simulink model "Vertical_rolling_Tongji_Control"  (R2021b)
settings: Solver=ode23s  StartTime=0.0  StopTime=7.5  FixedStep=1e-3  MaxStep=1e-3  RelTol=1e-3
values from neighbouring files (symbols this model uses):
  J_1 = m_1*r_1^2/2    (= 0.1)    [Vertical_Rolling_Tongji.m]
  J_2 = m_2*r_2^2/2    (= 2.5)    [Vertical_Rolling_Tongji.m]
  Klqr = lqr(sys,transpose(C)*Qu*C,R)    [Vertical_Rolling_Tongji.m]
  m_1 = 5    [Vertical_Rolling_Tongji.m]
  m_2 = 20    [Vertical_Rolling_Tongji.m]
  mu_d = 0.5    [Vertical_Rolling_Tongji.m]
  mu_r = mu_s*10^-2    (= 0.0065)    [Vertical_Rolling_Tongji.m]
  mu_s = 0.65    [Vertical_Rolling_Tongji.m]
  r_1 = 0.2    [Vertical_Rolling_Tongji.m]
  r_2 = 0.5    [Vertical_Rolling_Tongji.m]
  resolution = 5e-3    (= 0.005)    [Vertical_Rolling_Tongji.m]
  theta_1_0 = pi/3    (= 1.0471975512)    [Vertical_Rolling_Tongji.m]
libraries: simulink x1
settings Model: Creator=Gioele  LastModifiedBy=gioele
settings SolverCC: AlgebraicLoopSolver=TrustRegion
settings DebuggingCC: AlgebraicLoopMsg=none  SFMachineParentedDataDiag=warning

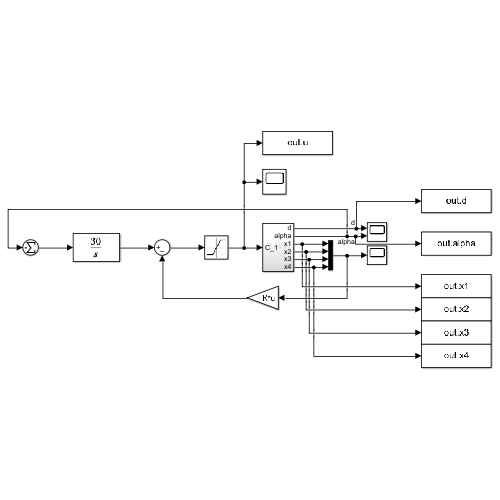
[thumbnail: Simulink's stored preview of the top-level diagram]
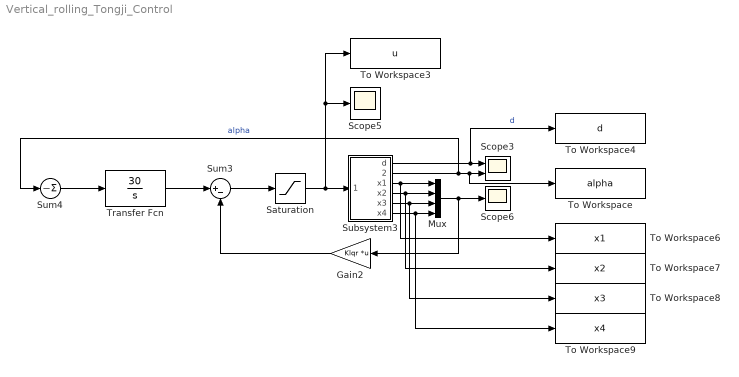
== system Vertical_rolling_Tongji_Control ==
  Gain2 : Gain  Gain=Klqr  Multiplication=Matrix(K*u)
  Mux : Mux
  Saturation : Saturate  UpperLimit=6  LowerLimit=-6
  Scope3 : Scope  NumInputPorts=2
  Scope5 : Scope
  Scope6 : Scope
  Subsystem3 : Subsystem
  Sum3 : Sum  Inputs=|+-
  Sum4 : Sum  Inputs=-
  To Workspace : ToWorkspace  VariableName=alpha  SampleTime=resolution
      settings: Save2DSignal=2-D array (concatenate along first dimension)
  To Workspace3 : ToWorkspace  VariableName=u  SampleTime=resolution
  To Workspace4 : ToWorkspace  VariableName=d  SampleTime=resolution
      settings: Save2DSignal=2-D array (concatenate along first dimension)
  To Workspace6 : ToWorkspace  VariableName=x1  SampleTime=-1
      settings: Save2DSignal=2-D array (concatenate along first dimension)
  To Workspace7 : ToWorkspace  VariableName=x2  SampleTime=-1
      settings: Save2DSignal=2-D array (concatenate along first dimension)
  To Workspace8 : ToWorkspace  VariableName=x3  SampleTime=-1
      settings: Save2DSignal=2-D array (concatenate along first dimension)
  To Workspace9 : ToWorkspace  VariableName=x4  SampleTime=-1
      settings: Save2DSignal=2-D array (concatenate along first dimension)
  Transfer Fcn : TransferFcn  Numerator=[30]  Denominator=[1 0]
  wires:
  Subsystem3/3(x1) -> To Workspace6/1, Mux/1
  Subsystem3/4(x2) -> Mux/2, To Workspace7/1
  Subsystem3/5(x3) -> Mux/3, To Workspace8/1
  Subsystem3/6(x4) -> Mux/4, To Workspace9/1
  Subsystem3/1(d) -> To Workspace4/1, Scope3/1  "d"
  Subsystem3/2(alpha) -> To Workspace/1, Scope3/2, Sum4/1  "alpha"
  Mux/1 -> Scope6/1, Gain2/1
  Gain2/1 -> Sum3/2
  Saturation/1 -> Subsystem3/1(C_1), To Workspace3/1, Scope5/1
  Sum3/1 -> Saturation/1
  Sum4/1 -> Transfer Fcn/1
  Transfer Fcn/1 -> Sum3/1

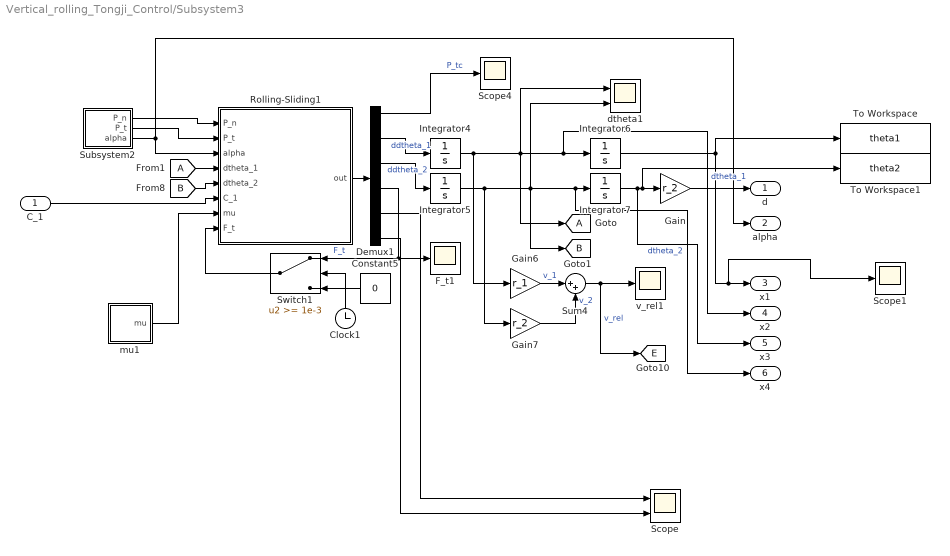
== system Vertical_rolling_Tongji_Control/Subsystem3 ==
  C_1 : Inport
  Clock1 : Clock
  Constant5 : Constant  Value=0
  Demux1 : Demux  Outputs=6
  F_t1 : Scope
  Gain : Gain  Gain=r_2
  Gain6 : Gain  Gain=r_1
  Gain7 : Gain  Gain=r_2
  Integrator4 : Integrator
  Integrator5 : Integrator
  Integrator6 : Integrator  InitialCondition=theta_1_0
  Integrator7 : Integrator
  Rolling-Sliding1 : MATLAB Function  TreatAsAtomicUnit=on
  Scope : Scope  NumInputPorts=2
  Scope1 : Scope
  Scope4 : Scope
  Subsystem2 : Subsystem
  Sum4 : Sum  Inputs=|++
  Switch1 : Switch  Threshold=1e-3  ZeroCross=off
  To Workspace : ToWorkspace  VariableName=theta1  SampleTime=resolution
  To Workspace1 : ToWorkspace  VariableName=theta2  SampleTime=resolution
  dtheta1 : Scope  NumInputPorts=2
  mu1 : Subsystem
  v_rel1 : Scope
  d : Outport
  alpha : Outport  Port=2
  x1 : Outport  Port=3
  x2 : Outport  Port=4
  x3 : Outport  Port=5
  x4 : Outport  Port=6
  tag scope: A=global, B=global, E=global
  wires:
  Subsystem2/2(P_t) -> Rolling-Sliding1/2(P_t)
  Integrator7/1 -> x3/1, To Workspace1/1, Gain/1
  Demux1/4 -> F_t1/1, Switch1/1  "F_t"
  mu1/1(mu) -> Rolling-Sliding1/7(mu)
  Integrator4/1 -> x2/1, Integrator6/1, [A], dtheta1/1, Gain6/1  "dtheta_1"
  Constant5/1 -> Switch1/3
  Gain6/1 -> Sum4/1  "v_1"
  [A] -> Rolling-Sliding1/4(dtheta_1)
  Clock1/1 -> Switch1/2
  Demux1/1 -> Scope4/1  "P_tc"
  Demux1/3 -> Integrator5/1  "ddtheta_2"
  Integrator5/1 -> Integrator7/1, x4/1, [B], dtheta1/2, Gain7/1  "dtheta_2"
  Subsystem2/1(P_n) -> Rolling-Sliding1/1(P_n)
  Demux1/2 -> Integrator4/1  "ddtheta_1"
  Switch1/1 -> Rolling-Sliding1/8(F_t)
  Integrator6/1 -> To Workspace/1, Scope1/1, x1/1
  Gain7/1 -> Sum4/2  "v_2"
  Rolling-Sliding1/1(out) -> Demux1/1
  Sum4/1 -> [E], v_rel1/1  "v_rel"
  [B] -> Rolling-Sliding1/5(dtheta_2)
  C_1/1 -> Rolling-Sliding1/6(C_1)
  Subsystem2/3(alpha) -> Rolling-Sliding1/3(alpha), alpha/1
  Gain/1 -> d/1
  Demux1/5 -> Scope/1
  Demux1/6 -> Scope/2

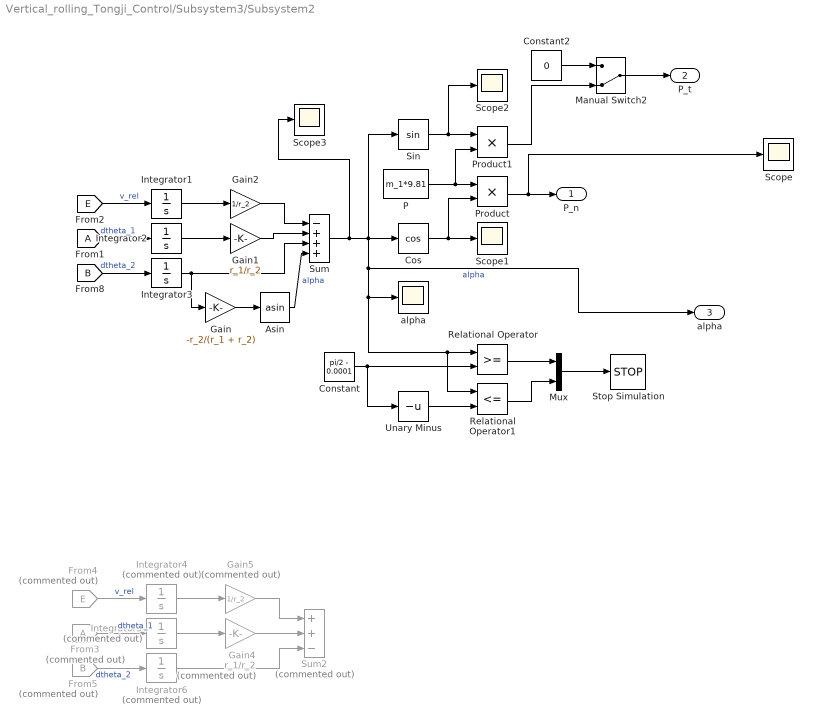
== system Vertical_rolling_Tongji_Control/Subsystem3/Subsystem2 ==
  Asin : Trigonometry  Operator=asin
  Constant : Constant  Value=pi/2 - 0.0001
  Constant2 : Constant  Value=0
  Cos : Trigonometry  Operator=cos
  From3 : From  Commented=on  TagVisibility=global
  From4 : From  Commented=on  GotoTag=E  TagVisibility=global
  From5 : From  Commented=on  GotoTag=B  TagVisibility=global
  Gain : Gain  Gain=-r_2/(r_1 + r_2)
  Gain1 : Gain  Gain=r_1/r_2
  Gain2 : Gain  Gain=1/r_2
  Gain4 : Gain  Commented=on  Gain=r_1/r_2
  Gain5 : Gain  Commented=on  Gain=1/r_2
  Integrator1 : Integrator
  Integrator2 : Integrator  InitialCondition=theta_1_0
  Integrator3 : Integrator
  Integrator4 : Integrator  Commented=on
  Integrator5 : Integrator  Commented=on  InitialCondition=theta_1_0
  Integrator6 : Integrator  Commented=on
  Manual Switch2 : ManualSwitch  CurrentSetting=0
  Mux : Mux  Inputs=2
  P : Constant  Value=m_1*9.81
  Product : Product
  Product1 : Product
  Relational Operator : RelationalOperator  OutDataTypeStr=boolean  RndMeth=Simplest
  Relational Operator1 : RelationalOperator  Operator=<=  OutDataTypeStr=boolean  RndMeth=Simplest
  Scope{,1..3} (4 alike) : Scope
  Sin : Trigonometry
  Stop Simulation : Stop
  Sum : Sum  Inputs=-+++
  Sum2 : Sum  Commented=on  Inputs=++-
  Unary Minus : UnaryMinus
  "alpha " : Scope
  P_n : Outport
  P_t : Outport  Port=2
  alpha : Outport  Port=3
  wires:
  P/1 -> Product1/2, Product/1
  [A] -> Integrator2/1  "dtheta_1"
  Integrator3/1 -> Sum/3, Gain/1
  Integrator2/1 -> Gain1/1
  [B] -> Integrator3/1  "dtheta_2"
  Product/1 -> Scope/1, P_n/1
  Gain1/1 -> Sum/2
  Cos/1 -> Scope1/1, Product/2
  [E] -> Integrator1/1  "v_rel"
  Integrator1/1 -> Gain2/1
  Gain2/1 -> Sum/1
  Constant/1 -> Unary Minus/1, Relational Operator/2
  Unary Minus/1 -> Relational Operator1/2
  Relational Operator/1 -> Mux/1
  Relational Operator1/1 -> Mux/2
  Mux/1 -> Stop Simulation/1
  Sin/1 -> Scope2/1, Product1/1
  Product1/1 -> Manual Switch2/2
  Constant2/1 -> Manual Switch2/1
  Manual Switch2/1 -> P_t/1
  From4/1 -> Integrator4/1  "v_rel"
  Integrator5/1 -> Gain4/1
  From3/1 -> Integrator5/1  "dtheta_1"
  Integrator6/1 -> Sum2/3
  From5/1 -> Integrator6/1  "dtheta_2"
  Gain4/1 -> Sum2/2
  Gain5/1 -> Sum2/1
  Integrator4/1 -> Gain5/1
  Sum/1 -> Scope3/1, Sin/1, Relational Operator1/1, Relational Operator/1, "alpha "/1, alpha/1, Cos/1  "alpha"
  Gain/1 -> Asin/1
  Asin/1 -> Sum/4  "alpha"

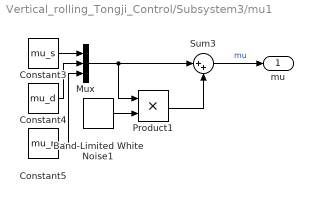
== system Vertical_rolling_Tongji_Control/Subsystem3/mu1 ==
  Band-Limited White Noise1 : simulink/Sources/Band-Limited White Noise  Cov=[0.000001]  Ts=0.1  seed=[23341]
  Constant3 : Constant  Value=mu_s
  Constant4 : Constant  Value=mu_d
  Constant5 : Constant  Value=mu_r
  Mux : Mux  Inputs=3
  Product1 : Product
  Sum3 : Sum  Inputs=|++
  mu : Outport
  wires:
  Sum3/1 -> mu/1  "mu"
  Constant5/1 -> Mux/3
  Constant4/1 -> Mux/2
  Product1/1 -> Sum3/2
  Constant3/1 -> Mux/1
  Mux/1 -> Sum3/1, Product1/1
  Band-Limited White Noise1/1 -> Product1/2

== matlab function Vertical_rolling_Tongji_Control/Subsystem3/Rolling-Sliding1 ==
  data: P_n input; P_t input; alpha input; dtheta_1 input; dtheta_2 input; C_1 input; r_1 parameter; r_2 parameter; J_1 parameter; J_2 parameter; mu input; F_t input; out output; m_2 parameter
function out = fcn(P_n,P_t,alpha,dtheta_1,dtheta_2,C_1,r_1,r_2,J_1,J_2,mu,F_t, m_2)
% Define the inputs of the function, some will be variables coming from the
% system, others will be parametsr from the workspace

mu_s_n = mu(1);
mu_d_n = mu(2);
mu_r_n = mu(3);
% Extract the values for the coefficients of friction from the white noise
% simulator

if abs(dtheta_1) > 0.01
    C_rf1 = - sign(dtheta_1)*mu_r_n*P_n;
else
%     if abs(C_1) < mu_r_n*P_n
%         C_rf1 = - C_1;
%     else
%         C_rf1 = - sign(dtheta_1)*mu_r_n*P_n;
%     end
    C_rf1 = 0;
end
% C_rf1 = - sign(dtheta_1)*mu_r_n*P_n;
if abs(dtheta_2) > 0.01
    C_rf2 = - sign(dtheta_2)*mu_r_n*P_n;
else
%     if abs(- F_t*r_2) < mu_r_n*P_n
%         C_rf2 = - (- F_t*r_2);
%     else
%         C_rf2 = - sign(dtheta_2)*mu_r_n*P_n;
%     end
    C_rf2 = 0;
end
% C_rf2 = - sign(dtheta_2)*mu_r_n*P_n;
% Define the action of the rolling friction forces C_rf1 and C_rf2

if (-0.0001 < dtheta_1*r_1 + dtheta_2*r_2) && (dtheta_1*r_1 + dtheta_2*r_2 < 0.0001)
    % Condition should be (dtheta_1*r_1 + dtheta_2*r_2 == 0) but need
    % tolerance for simulation reasons
    P_tc = P_t;
    F_t = (C_1*(r_1/J_1) + C_rf1*(r_1/J_1) + C_rf2*(r_2/J_2) - P_tc*(r_1^2/J_1) - P_tc*(r_2^2/J_2) - P_n*sin(alpha)*(r_2^2/(J_2+m_2*r_2^2)))/((r_1^2/J_1) + (r_2^2/J_2));
    % Define the two tangential forces P_tc and F_t in the pure rolling
    % case
    if (abs(F_t + P_tc) > mu_s_n*P_n)
        P_tc = sign(alpha)*mu_d_n*P_n;
        F_t = sign(dtheta_1*r_1 + dtheta_2*r_2)*mu_d_n*P_n;
        % Transition from Rolling to Rolling with sliding
    end
else
    P_tc = sign(alpha)*mu_d_n*P_n;
    F_t = sign(dtheta_1*r_1 + dtheta_2*r_2)*mu_d_n*P_n;
    % Define the two tangential forces P_tc and F_t in the pure rolling
    % case
end

ddtheta_1 = (C_1 + C_rf1 - F_t*r_1 - P_tc*r_1)/(J_1);
ddtheta_2 = ((- F_t*r_2 - P_tc*r_2 + C_rf2 )/(J_2))-((P_n*sin(alpha)*r_2)/(J_2+m_2*r_2^2));
% Get out the final expression for the two angular speeds

out = [P_tc,ddtheta_1,ddtheta_2,F_t,C_rf1,C_rf2];
% Define the outputs of the system
